simulink model "CrCtl_ShOff"  (R2016b)
settings: configuration reference "CodeGenConfigSet" (kept outside this file)
values from neighbouring files (symbols this model uses):
  CrCtl_aAccShOff_C = Calibration.Parameter    [init_CrCtl_ShOff.m]
  CrCtl_aDeclShOff_C = Calibration.Parameter    [init_CrCtl_ShOff.m]
  CrCtl_facDvtRelShOff_C = Calibration.Parameter    [init_CrCtl_ShOff.m]
  CrCtl_GearMin_C = Calibration.Parameter    [init_CrCtl_ShOff.m]
  CrCtl_nMaxShOff_C = Calibration.Parameter    [init_CrCtl_ShOff.m]
  CrCtl_nMinShOff_C = Calibration.Parameter    [init_CrCtl_ShOff.m]
  CRCTL_PAUSEENABLE_SY = uint8(0)    [init_CrCtl_ShOff.m]
  CrCtl_rTraV2NDvtAbsShOff_C = Calibration.Parameter    [init_CrCtl_ShOff.m]
  CrCtl_rTraV2NDvtShOff_C = Calibration.Parameter    [init_CrCtl_ShOff.m]
  CrCtl_rTraV2NSuspSync_C = Calibration.Parameter    [init_CrCtl_ShOff.m]
  CrCtl_stShOffCut_C = Calibration.Parameter    [init_CrCtl_ShOff.m]
  CrCtl_stShOffIrvrs_C = Calibration.Parameter    [init_CrCtl_ShOff.m]
  CrCtl_stShOffRvrs_C = Calibration.Parameter    [init_CrCtl_ShOff.m]
  CrCtl_stShOffRvrsDelVel_C = Calibration.Parameter    [init_CrCtl_ShOff.m]
  CrCtl_stShOffSlpCnstRmp_C = Calibration.Parameter    [init_CrCtl_ShOff.m]
  CrCtl_stShOffTimeCnstRmp_C = Calibration.Parameter    [init_CrCtl_ShOff.m]
  CrCtl_swtSuspEna_C = Calibration.Parameter    [init_CrCtl_ShOff.m]
  CrCtl_tiAccShOff_C = Calibration.Parameter    [init_CrCtl_ShOff.m]
  CrCtl_tiDeclShOff_C = Calibration.Parameter    [init_CrCtl_ShOff.m]
  CrCtl_tiDvtShOff_C = Calibration.Parameter    [init_CrCtl_ShOff.m]
  CrCtl_tiOverrideShOff_C = Calibration.Parameter    [init_CrCtl_ShOff.m]
  CrCtl_tiSuspClthPresMax_C = Calibration.Parameter    [init_CrCtl_ShOff.m]
  CrCtl_tiSuspMax_C = Calibration.Parameter    [init_CrCtl_ShOff.m]
  CrCtl_tiSuspSync_C = Calibration.Parameter    [init_CrCtl_ShOff.m]
  CrCtl_trqSpdGovInc_C = Calibration.Parameter    [init_CrCtl_ShOff.m]
  CrCtl_trqSpdGovMax_C = Calibration.Parameter    [init_CrCtl_ShOff.m]
  CrCtl_trqSpdGovRed_C = Calibration.Parameter    [init_CrCtl_ShOff.m]
  CrCtl_vDvtNegShOff_C = Calibration.Parameter    [init_CrCtl_ShOff.m]
  CrCtl_vDvtPosShOff_C = Calibration.Parameter    [init_CrCtl_ShOff.m]
  CrCtl_vDvtShOff_C = Calibration.Parameter    [init_CrCtl_ShOff.m]
  CrCtl_vMaxShOff_C = Calibration.Parameter    [init_CrCtl_ShOff.m]
  CrCtl_vMinShOff_C = Calibration.Parameter    [init_CrCtl_ShOff.m]
  TRQ_ENGINTV_SY = uint8(1)    [init_CrCtl_ShOff.m]
  VEL_ZERO = fi(0,VehSpeed_km_h)    [init_CrCtl_ShOff.m]
undefined symbols (not defined in the file or in its folder): CrCtl_ShOff_DT, CrCtl_stLck_conv, CrCtl_stOpFunc_conv, CrCtl_stShOff_conv, CrCtl_stSub_conv, CrCUI_BttnState_conv, CruiseCtl_State_conv, EngState_conv, Switch_conv
libraries: simulink x80, CXLib x24
(part 1 of 2)
settings Model: Creator=guanxiaoxing  LastModifiedBy=guanxiaoxing
settings ConfigSetRef: SourceLocation=Base Workspace

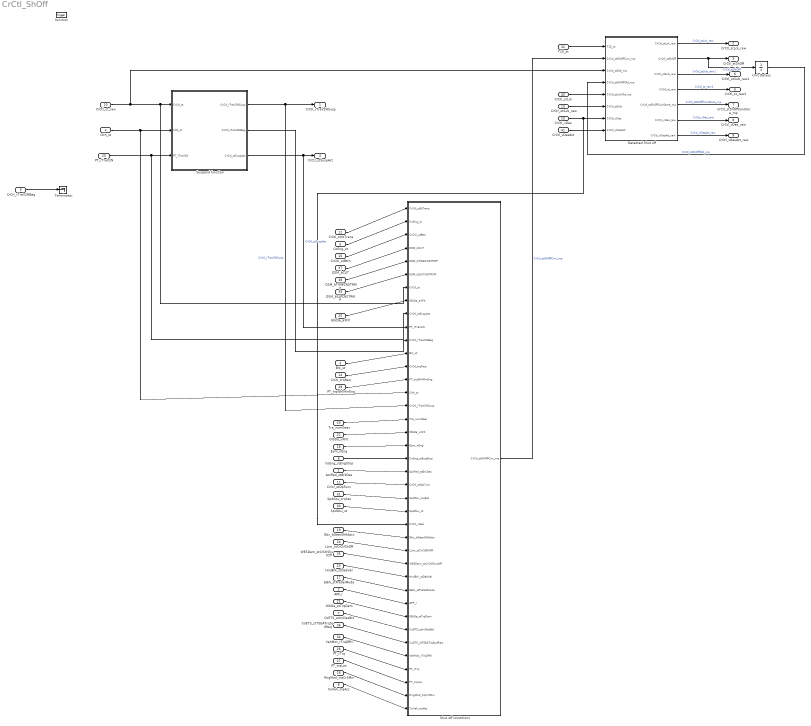
== system CrCtl_ShOff ==
  AccPed_stBrkDes : Inport  Description=Application parameter for engine brake request  OutMin=0  OutMax=255  OutDataTypeStr=State_uint8
  APP_r : Inport  Tag=%  Description=Acceleration pedal sensor 1 value after fault handling  Port=2  OutMin=0  OutMax=100  OutDataTypeStr=Accpedal_rate
  Brk_st : Inport  Description=Brake switch state  Port=3  OutMin=0  OutMax=255  OutDataTypeStr=State_uint8
  Clth_st : Inport  Description=Clutch information  Port=4  OutMin=0  OutMax=255  OutDataTypeStr=State_uint8
  CoEng_st : Inport  Description=Engine coordinator state  Port=5  OutDataTypeStr=Enum: EngState_conv
  CoEng_stEngStop : Inport  Description=Bit coded output message from engine stop function for low idle, egine shut off and crank control  Port=6  OutMin=0  OutMax=255  OutDataTypeStr=State_uint8
  CoETS_stInrDesBrk : Inport  Description=Negative torque status for inner torque  Port=7  OutMin=0  OutMax=4294967295  OutDataTypeStr=State_uint32
  CoVeh_trqAcs : Inport  Tag=Nm  Description=message for torque demand of accessories  Port=8  OutMin=-3276.8  OutMax=3276.7  OutDataTypeStr=Trq_Nm
  CrCtl_rTraV2NBeg : Inport  Tag=km/h/rpm  Description=V/N ratio at activation of cruise control  Port=9  OutMin=-0.32768  OutMax=0.32767  OutDataTypeStr=Tra_V2N_km_h_rpm
  CrCtl_st_raw : Inport  Description=Application parameter for Cruise Control state  Port=10  OutDataTypeStr=Enum: CruiseCtl_State_conv
  CrCtl_stOpFunc : Inport  Description=state of cruise control operation functionality  Port=11  OutDataTypeStr=Enum: CrCtl_stOpFunc_conv
  CrCtl_stStTrans : Inport  Description=|  Port=12  OutDataTypeStr=Enum: CrCUI_BttnState_conv
      | State transition demand to the state machine of
      | cruise control
  CrCtl_stSub_raw : Inport  Description=Cruise control sub mode  Port=13  OutDataTypeStr=Enum: CrCtl_stSub_conv
  CrCtl_trqReq : Inport  Tag=Nm  Description=Cruise control torque request  Port=14  OutMin=-3000  OutMax=3000  OutDataTypeStr=Trq_Nm
  CrCtl_vDes : Inport  Tag=km/h  Description=Cruise Control desired set point speed  Port=15  OutMin=0  OutMax=250  OutDataTypeStr=VehSpeed_km_h
  CrCUI_stBttn : Inport  Description=Application parameter for status button information  Port=16  OutDataTypeStr=Enum: CrCUI_BttnState_conv
  EBrk_stPreSelMode : Inport  Description=Status of Engine Brake Pre-Selection modes  Port=17  OutDataTypeStr=Enum: EBrk_stPreSelMode_conv
  Epm_nEng : Inport  Tag=rpm  Description=Engine speed  Port=18  OutMin=0  OutMax=6000  OutDataTypeStr=EngSpeed_rpm
  Gbx_bGearShftActv : Inport  Description=Status gear shift active  Port=19  OutMin=0  OutMax=1  OutDataTypeStr=boolean
  GlbDa_aXFlt : Inport  Tag=m/s^2  Description=Vehicle longitudinal acceleration filtered  Port=20  OutMin=-32  OutMax=32  OutDataTypeStr=Acc_m_s2
  GlbDa_stTrqDem : Inport  Description=Contains highest prior function with torque demand  Port=21  OutMin=0  OutMax=4294967295  OutDataTypeStr=State_uint32
  GlbDa_vXFlt : Inport  Tag=km/h  Description=Vehicle velocity filtered  Port=22  OutMin=0  OutMax=250  OutDataTypeStr=VehSpeed_km_h
  HndBrk_stDebVal : Inport  Description=Debounced value of Hand Brake switch  Port=23  OutMin=0  OutMax=255  OutDataTypeStr=State_uint8
  LLim_stCrCtlShOff : Inport  Description=shutoff request for cruise control  Port=24  OutMin=0  OutMax=1  OutDataTypeStr=boolean
  PT_rTraV2N : Inport  Tag=km/h/rpm  Description=Quotient of velocity and engine speed  Port=25  OutMin=-0.32768  OutMax=0.32767  OutDataTypeStr=Tra_V2N_km_h_rpm
  PT_rTrq : Inport  Description=Powertrain torque ratio  Port=26  OutMin=-100  OutMax=100  OutDataTypeStr=TransRatio
  PT_trqLos : Inport  Tag=Nm  Description=Parameter for loss torque of the drive train  Port=27  OutMin=-3000  OutMax=3000  OutDataTypeStr=Trq_Nm
  PT_trqWhlMinEng : Inport  Tag=Nm  Description=Minimum wheel torque from the engine  Port=28  OutMin=-3000  OutMax=3000  OutDataTypeStr=Trq_Nm
  RngMod_trqCrSMin : Inport  Tag=Nm  Description=Minimal crankshaft torque  Port=29  OutMin=-3276.8  OutMax=3276.7  OutDataTypeStr=Trq_Nm
  SpdGov_st : Inport  Description=Status speed control SpdGov  Port=30  OutMin=0  OutMax=65535  OutDataTypeStr=State_uint16
  SpdGov_trqSet : Inport  Tag=Nm  Description=Set point torque of the SpdGov on the fuel path  Port=31  OutMin=-3000  OutMax=3000  OutDataTypeStr=Trq_Nm
  T15_st : Inport  Description=Terminal 15 status after denouncing  Port=32  OutDataTypeStr=Enum: Switch_conv
  Tra_numGear : Inport  Description=Current gear information  Port=33  OutMin=-128  OutMax=127  OutDataTypeStr=Tra_num
  VehMot_rTrqDfftl : Inport  Description=Torque ratio of differential  Port=34  OutMin=-300  OutMax=300  OutDataTypeStr=TransRatio
  WESDem_stCrCtlShutOff : Inport  Description=Shut off of the cruise control  Port=35  OutMin=0  OutMax=1  OutDataTypeStr=boolean
  CoETS_stTSEATrqSpdReq : Inport  Description=Status of information about torque and speed intervention  Port=36  OutMin=0  OutMax=65535  OutDataTypeStr=State_uint16
  DSM_bCUT : Inport  Description=status of Fid_CUT  Port=37  OutMin=0  OutMax=1  OutDataTypeStr=boolean
  DSM_bTIMECNSTRMP : Inport  Description=status of Fid_TIMECNSTRMP  Port=38  OutMin=0  OutMax=1  OutDataTypeStr=boolean
  DSM_bSLPCNSTRMP : Inport  Description=status of Fid_SLPCNSTRMP  Port=39  OutMin=0  OutMax=1  OutDataTypeStr=boolean
  CrCtl_stLck : Inport  Description=Cruise Control lock Status  Port=40  OutDataTypeStr=Enum: CrCtl_stLck_conv
  CrCtl_vDesAct : Inport  Tag=km/h  Description=Target speed for cruise control  Port=41  OutMin=0  OutMax=250  OutDataTypeStr=VehSpeed_km_h
  function : TriggerPort  TriggerType=function-call  VariantControl=Variant
  Detected Shut off : Subsystem
  Shut off conditions : Subsystem
  Suspend function : Subsystem
  Terminator : Terminator
  Unit Delay1 : UnitDelay  InitialCondition=CrCtl_stShOff_conv.CRCTL_NOSHOFFCONACTV  SampleTime=-1
  CrCtl_rTraV2NSusp : Outport  Tag=km/h/rpm  Description=V/N ratio for the pressed clutch during active Suspend mode  OutMin=-0.32768  OutMax=0.32767  OutDataTypeStr=Tra_V2N_km_h_rpm
  CrCtl_stLck_raw : Outport  Description=Cruise Control lock Status  Port=2  OutDataTypeStr=Enum: CrCtl_stLck_conv
  CrCtl_stShOff : Outport  Description=cruise control shut-off requirement  Port=3  OutDataTypeStr=Enum: CrCtl_stShOff_conv
  CrCtl_stSuspAct : Outport  Description=Cruise Control suspend mode active Status  Port=4  OutMin=0  OutMax=1  OutDataTypeStr=boolean
  CrCtl_st_raw1 : Outport  Description=Application parameter for Cruise Control state  Port=5  OutDataTypeStr=Enum: CruiseCtl_State_conv
  CrCtl_stSub_raw1 : Outport  Description=Cruise control sub mode  Port=6  OutDataTypeStr=Enum: CrCtl_stSub_conv
  CrCtl_stShOffConStore_mp : Outport  Description=Status of Shutoff condition  Port=7  OutMin=0  OutMax=4294967295  OutDataTypeStr=State_uint32
  CrCtl_vDes_raw : Outport  Tag=km/h  Description=Cruise Control desired set point speed  Port=8  OutMin=0  OutMax=250  OutDataTypeStr=VehSpeed_km_h
  CrCtl_vDesAct_raw : Outport  Tag=km/h  Description=Target speed for cruise control  Port=9  OutMin=0  OutMax=250  OutDataTypeStr=VehSpeed_km_h
  wires:
  Suspend function/1(CrCtl_rTraV2NSusp) -> CrCtl_rTraV2NSusp/1, Shut off conditions/16(CrCtl_rTraV2NSusp)  "CrCtl_rTraV2NSusp"
  Detected Shut off/1(CrCtl_stLck_raw) -> CrCtl_stLck_raw/1  "CrCtl_stLck_raw"
  Detected Shut off/2(CrCtl_stShOff) -> Unit Delay1/1, CrCtl_stShOff/1  "CrCtl_stShOff"
  Suspend function/3(CrCtl_stSuspAct) -> CrCtl_stSuspAct/1, Shut off conditions/9(CrCtl_stSuspAct)  "CrCtl_stSuspAct"
  T15_st/1 -> Detected Shut off/1(T15_st)
  CrCtl_st_raw/1 -> Shut off conditions/7(CrCtl_st), Suspend function/1(CrCtl_st), Detected Shut off/3(CrCtl_stOld_mp)
  Shut off conditions/1(CrCtl_stShOffCon_mp) -> Detected Shut off/2(CrCtl_stShOffCon_mp)  "CrCtl_stShOffCon_mp"
  Unit Delay1/1 -> Detected Shut off/4(CrCtl_stShOffOld_mp)  "CrCtl_stShOffOld_mp"
  CrCtl_stStTrans/1 -> Shut off conditions/1(CrCtl_stStTrans)
  CoEng_st/1 -> Shut off conditions/2(CoEng_st)
  CrCUI_stBttn/1 -> Shut off conditions/3(CrCUI_stBttn)
  GlbDa_aXFlt/1 -> Shut off conditions/8(GlbDa_aXFlt)
  PT_rTraV2N/1 -> Suspend function/3(PT_rTraV2N), Shut off conditions/10(PT_rTraV2N)
  Suspend function/2(CrCtl_rTraV2NBeg) -> Shut off conditions/11(CrCtl_rTraV2NBeg)
  Brk_st/1 -> Shut off conditions/12(Brk_st)
  CrCtl_trqReq/1 -> Shut off conditions/13(CrCtl_trqReq)
  PT_trqWhlMinEng/1 -> Shut off conditions/14(PT_trqWhlMinEng)
  Clth_st/1 -> Shut off conditions/15(Clth_st), Suspend function/2(Clth_st)
  Tra_numGear/1 -> Shut off conditions/17(Tra_numGear)
  GlbDa_vXFlt/1 -> Shut off conditions/18(GlbDa_vXFlt)
  Epm_nEng/1 -> Shut off conditions/19(Epm_nEng)
  CoEng_stEngStop/1 -> Shut off conditions/20(CoEng_stEngStop)
  AccPed_stBrkDes/1 -> Shut off conditions/21(AccPed_stBrkDes)
  CrCtl_stOpFunc/1 -> Shut off conditions/22(CrCtl_stOpFunc)
  SpdGov_trqSet/1 -> Shut off conditions/23(SpdGov_trqSet)
  SpdGov_st/1 -> Shut off conditions/24(SpdGov_st)
  CrCtl_vDes/1 -> Shut off conditions/25(CrCtl_vDes), Detected Shut off/7(CrCtl_vDes)
  Gbx_bGearShftActv/1 -> Shut off conditions/26(Gbx_bGearShftActv)
  LLim_stCrCtlShOff/1 -> Shut off conditions/27(LLim_stCrCtlShOff)
  WESDem_stCrCtlShutOff/1 -> Shut off conditions/28(WESDem_stCrCtlShutOff)
  HndBrk_stDebVal/1 -> Shut off conditions/29(HndBrk_stDebVal)
  CoETS_stTSEATrqSpdReq/1 -> Shut off conditions/34(CoETS_stTSEATrqSpdReq)
  EBrk_stPreSelMode/1 -> Shut off conditions/30(EBrk_stPreSelMode)
  APP_r/1 -> Shut off conditions/31(APP_r)
  PT_rTrq/1 -> Shut off conditions/36(PT_rTrq)
  PT_trqLos/1 -> Shut off conditions/37(PT_trqLos)
  RngMod_trqCrSMin/1 -> Shut off conditions/38(RngMod_trqCrSMin)
  CoVeh_trqAcs/1 -> Shut off conditions/39(CoVeh_trqAcs)
  VehMot_rTrqDfftl/1 -> Shut off conditions/35(VehMot_rTrqDfftl)
  CoETS_stInrDesBrk/1 -> Shut off conditions/33(CoETS_stInrDesBrk)
  GlbDa_stTrqDem/1 -> Shut off conditions/32(GlbDa_stTrqDem)
  DSM_bCUT/1 -> Shut off conditions/4(DSM_bCUT)
  DSM_bTIMECNSTRMP/1 -> Shut off conditions/5(DSM_bTIMECNSTRMP)
  DSM_bSLPCNSTRMP/1 -> Shut off conditions/6(DSM_bSLPCNSTRMP)
  CrCtl_stSub_raw/1 -> Detected Shut off/6(CrCtl_stSub)
  Detected Shut off/5(CrCtl_stShOffConStore_mp) -> CrCtl_stShOffConStore_mp/1  "CrCtl_stShOffConStore_mp"
  CrCtl_rTraV2NBeg/1 -> Terminator/1
  CrCtl_stLck/1 -> Detected Shut off/5(CrCtl_stLckOld_mp)
  Detected Shut off/6(CrCtl_vDes_raw) -> CrCtl_vDes_raw/1  "CrCtl_vDes_raw"
  Detected Shut off/7(CrCtl_vDesAct_raw) -> CrCtl_vDesAct_raw/1  "CrCtl_vDesAct_raw"
  CrCtl_vDesAct/1 -> Detected Shut off/8(CrCtl_vDesAct)
  Detected Shut off/3(CrCtl_stSub_raw) -> CrCtl_stSub_raw1/1  "CrCtl_stSub_raw1"
  Detected Shut off/4(CrCtl_st_raw) -> CrCtl_st_raw1/1  "CrCtl_st_raw1"

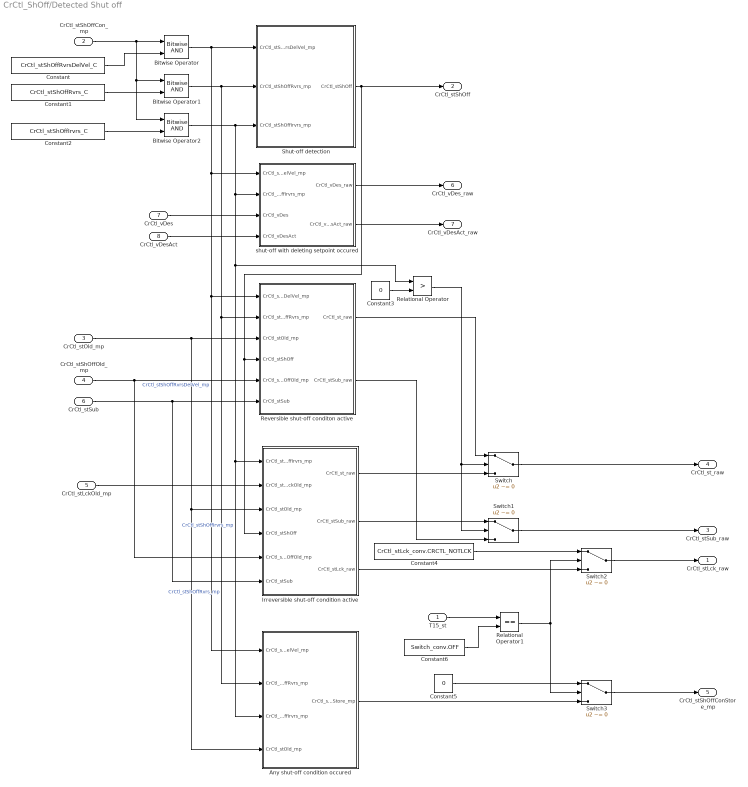
== system CrCtl_ShOff/Detected Shut off ==
  T15_st : Inport
  CrCtl_stShOffCon_mp : Inport  Port=2
  CrCtl_stOld_mp : Inport  Port=3
  CrCtl_stShOffOld_mp : Inport  Port=4
  CrCtl_stLckOld_mp : Inport  Port=5
  CrCtl_stSub : Inport  Port=6
  CrCtl_vDes : Inport  Port=7
  CrCtl_vDesAct : Inport  Port=8
  Any shut-off condition occured : Subsystem
  Bitwise Operator : simulink/Logic and Bit Operations/Bitwise Operator  logicop=AND  UseBitMask=off  NumInputPorts=2  BitMask=bin2dec('11011001')  BitMaskRealWorld=Stored Integer
  Bitwise Operator1 : simulink/Logic and Bit Operations/Bitwise Operator  logicop=AND  UseBitMask=off  NumInputPorts=2  BitMask=bin2dec('11011001')  BitMaskRealWorld=Stored Integer
  Bitwise Operator2 : simulink/Logic and Bit Operations/Bitwise Operator  logicop=AND  UseBitMask=off  NumInputPorts=2  BitMask=bin2dec('11011001')  BitMaskRealWorld=Stored Integer
  Constant : Constant  Value=CrCtl_stShOffRvrsDelVel_C
  Constant1 : Constant  Value=CrCtl_stShOffRvrs_C
  Constant2 : Constant  Value=CrCtl_stShOffIrvrs_C
  Constant3 : Constant  Value=0
  Constant4 : Constant  Value=CrCtl_stLck_conv.CRCTL_NOTLCK
  Constant5 : Constant  Value=0  OutDataTypeStr=uint16
  Constant6 : Constant  Value=Switch_conv.OFF
  Irreversible shut-off condition active : Subsystem
  Relational Operator : RelationalOperator  Operator=>  OutDataTypeStr=boolean  RndMeth=Simplest
  Relational Operator1 : RelationalOperator  Operator===  OutDataTypeStr=boolean  RndMeth=Simplest
  Reversible shut-off conditon active : Subsystem
  Shut-off detection : Subsystem
  Switch{,1..3} (4 alike) : Switch  Criteria=u2 ~= 0
  shut-off with deleting setpoint occured : Subsystem
  CrCtl_stLck_raw : Outport
  CrCtl_stShOff : Outport  Port=2
  CrCtl_stSub_raw : Outport  Port=3
  CrCtl_st_raw : Outport  Port=4
  CrCtl_stShOffConStore_mp : Outport  Port=5
  CrCtl_vDes_raw : Outport  Port=6
  CrCtl_vDesAct_raw : Outport  Port=7
  wires:
  CrCtl_stShOffCon_mp/1 -> Bitwise Operator2/1, Bitwise Operator1/1, Bitwise Operator/1
  Constant/1 -> Bitwise Operator/2
  Constant1/1 -> Bitwise Operator1/2
  Constant2/1 -> Bitwise Operator2/2
  Bitwise Operator/1 -> Shut-off detection/1(CrCtl_stShOffRvrsDelVel_mp), Any shut-off condition occured/1(CrCtl_stShOffRvrsDelVel_mp), Reversible shut-off conditon active/1(CrCtl_stShOffRvrsDelVel_mp), shut-off with deleting setpoint occured/1(CrCtl_stShOffRvrsDelVel_mp)  "CrCtl_stShOffRvrsDelVel_mp"
  Bitwise Operator1/1 -> Any shut-off condition occured/2(CrCtl_stShOffRvrs_mp), Reversible shut-off conditon active/2(CrCtl_stShOffRvrs_mp), Shut-off detection/2(CrCtl_stShOffRvrs_mp)  "CrCtl_stShOffRvrs_mp"
  Bitwise Operator2/1 -> Relational Operator/1, Irreversible shut-off condition active/1(CrCtl_stShOffIrvrs_mp), Any shut-off condition occured/3(CrCtl_stShOffIrvrs_mp), shut-off with deleting setpoint occured/2(CrCtl_stShOffIrvrs_mp), Shut-off detection/3(CrCtl_stShOffIrvrs_mp)  "CrCtl_stShOffIrvrs_mp"
  Constant3/1 -> Relational Operator/2
  CrCtl_stOld_mp/1 -> Any shut-off condition occured/4(CrCtl_stOld_mp), Irreversible shut-off condition active/3(CrCtl_stOld_mp), Reversible shut-off conditon active/3(CrCtl_stOld_mp)
  CrCtl_stShOffOld_mp/1 -> Irreversible shut-off condition active/5(CrCtl_stShOffOld_mp), Reversible shut-off conditon active/5(CrCtl_stShOffOld_mp)
  Reversible shut-off conditon active/1(CrCtl_st_raw) -> Switch/1
  Relational Operator/1 -> Switch/2, Switch1/2
  Irreversible shut-off condition active/1(CrCtl_st_raw) -> Switch/3
  Reversible shut-off conditon active/2(CrCtl_stSub_raw) -> Switch1/3
  Irreversible shut-off condition active/3(CrCtl_stLck_raw) -> Switch2/3
  Irreversible shut-off condition active/2(CrCtl_stSub_raw) -> Switch1/1
  Relational Operator1/1 -> Switch3/2, Switch2/2
  Constant4/1 -> Switch2/1
  Any shut-off condition occured/1(CrCtl_stShOffConStore_mp) -> Switch3/3
  Constant5/1 -> Switch3/1
  Switch1/1 -> CrCtl_stSub_raw/1
  Switch/1 -> CrCtl_st_raw/1
  Switch3/1 -> CrCtl_stShOffConStore_mp/1
  shut-off with deleting setpoint occured/1(CrCtl_vDes_raw) -> CrCtl_vDes_raw/1
  Switch2/1 -> CrCtl_stLck_raw/1
  Shut-off detection/1(CrCtl_stShOff) -> CrCtl_stShOff/1, Irreversible shut-off condition active/4(CrCtl_stShOff), Reversible shut-off conditon active/4(CrCtl_stShOff)
  CrCtl_stSub/1 -> Irreversible shut-off condition active/6(CrCtl_stSub), Reversible shut-off conditon active/6(CrCtl_stSub)
  CrCtl_stLckOld_mp/1 -> Irreversible shut-off condition active/2(CrCtl_stLckOld_mp)
  CrCtl_vDes/1 -> shut-off with deleting setpoint occured/3(CrCtl_vDes)
  shut-off with deleting setpoint occured/2(CrCtl_vDesAct_raw) -> CrCtl_vDesAct_raw/1
  CrCtl_vDesAct/1 -> shut-off with deleting setpoint occured/4(CrCtl_vDesAct)
  T15_st/1 -> Relational Operator1/1
  Constant6/1 -> Relational Operator1/2

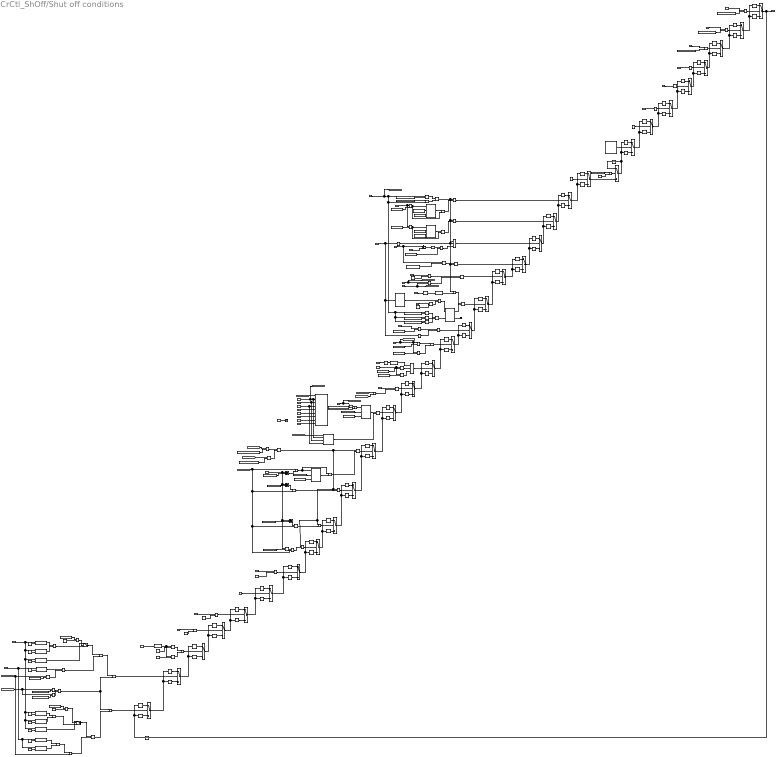
== system CrCtl_ShOff/Shut off conditions ==
  CrCtl_stStTrans : Inport
  CoEng_st : Inport  Port=2
  CrCUI_stBttn : Inport  Port=3
  DSM_bCUT : Inport  Port=4
  DSM_bTIMECNSTRMP : Inport  Port=5
  DSM_bSLPCNSTRMP : Inport  Port=6
  CrCtl_st : Inport  Port=7
  GlbDa_aXFlt : Inport  Port=8
  CrCtl_stSuspAct : Inport  Port=9
  PT_rTraV2N : Inport  Port=10
  CrCtl_rTraV2NBeg : Inport  Port=11
  Brk_st : Inport  Port=12
  CrCtl_trqReq : Inport  Port=13
  PT_trqWhlMinEng : Inport  Port=14
  Clth_st : Inport  Port=15
  CrCtl_rTraV2NSusp : Inport  Port=16
  Tra_numGear : Inport  Port=17
  GlbDa_vXFlt : Inport  Port=18
  Epm_nEng : Inport  Port=19
  CoEng_stEngStop : Inport  Port=20
  AccPed_stBrkDes : Inport  Port=21
  CrCtl_stOpFunc : Inport  Port=22
  SpdGov_trqSet : Inport  Port=23
  SpdGov_st : Inport  Port=24
  CrCtl_vDes : Inport  Port=25
  Gbx_bGearShftActv : Inport  Port=26
  LLim_stCrCtlShOff : Inport  Port=27
  WESDem_stCrCtlShutOff : Inport  Port=28
  HndBrk_stDebVal : Inport  Port=29
  EBrk_stPreSelMode : Inport  Port=30
  APP_r : Inport  Port=31
  GlbDa_stTrqDem : Inport  Port=32
  CoETS_stInrDesBrk : Inport  Port=33
  CoETS_stTSEATrqSpdReq : Inport  Port=34
  VehMot_rTrqDfftl : Inport  Port=35
  PT_rTrq : Inport  Port=36
  PT_trqLos : Inport  Port=37
  RngMod_trqCrSMin : Inport  Port=38
  CoVeh_trqAcs : Inport  Port=39
  Abs : Abs
  Add : Sum  Inputs=+-
  Add1 : Sum
  Add2 : Sum
  Add3 : Sum  Inputs=+-
  Bit Clear : simulink/Logic and Bit Operations/Bit Clear  iBit=0
  Bit Clear1 : simulink/Logic and Bit Operations/Bit Clear  iBit=1
  Bit Clear10 : simulink/Logic and Bit Operations/Bit Clear  iBit=11
  Bit Clear11 : simulink/Logic and Bit Operations/Bit Clear  iBit=12
  Bit Clear12 : simulink/Logic and Bit Operations/Bit Clear  iBit=13
  Bit Clear13 : simulink/Logic and Bit Operations/Bit Clear  iBit=14
  Bit Clear14 : simulink/Logic and Bit Operations/Bit Clear  iBit=15
  Bit Clear15 : simulink/Logic and Bit Operations/Bit Clear  iBit=16
  Bit Clear16 : simulink/Logic and Bit Operations/Bit Clear  iBit=17
  Bit Clear17 : simulink/Logic and Bit Operations/Bit Clear  iBit=18
  Bit Clear18 : simulink/Logic and Bit Operations/Bit Clear  iBit=19
  Bit Clear19 : simulink/Logic and Bit Operations/Bit Clear  iBit=20
  Bit Clear2 : simulink/Logic and Bit Operations/Bit Clear  iBit=2
  Bit Clear20 : simulink/Logic and Bit Operations/Bit Clear  iBit=21
  Bit Clear21 : simulink/Logic and Bit Operations/Bit Clear  iBit=22
  Bit Clear22 : simulink/Logic and Bit Operations/Bit Clear  iBit=23
  Bit Clear23 : simulink/Logic and Bit Operations/Bit Clear  iBit=24
  Bit Clear24 : simulink/Logic and Bit Operations/Bit Clear  iBit=25
  Bit Clear25 : simulink/Logic and Bit Operations/Bit Clear  iBit=26
  Bit Clear26 : simulink/Logic and Bit Operations/Bit Clear  iBit=27
  Bit Clear27 : simulink/Logic and Bit Operations/Bit Clear  iBit=28
  Bit Clear28 : simulink/Logic and Bit Operations/Bit Clear  iBit=29
  Bit Clear29 : simulink/Logic and Bit Operations/Bit Clear  iBit=30
  Bit Clear3 : simulink/Logic and Bit Operations/Bit Clear  iBit=3
  Bit Clear30 : simulink/Logic and Bit Operations/Bit Clear  iBit=31
  Bit Clear4 : simulink/Logic and Bit Operations/Bit Clear  iBit=4
  Bit Clear5 : simulink/Logic and Bit Operations/Bit Clear  iBit=5
  Bit Clear6 : simulink/Logic and Bit Operations/Bit Clear  iBit=6
  Bit Clear7 : simulink/Logic and Bit Operations/Bit Clear  iBit=7
  Bit Clear8 : simulink/Logic and Bit Operations/Bit Clear  iBit=8
  Bit Clear9 : simulink/Logic and Bit Operations/Bit Clear  iBit=10
  Bit Set : simulink/Logic and Bit Operations/Bit Set  iBit=0
  Bit Set1 : simulink/Logic and Bit Operations/Bit Set  iBit=1
  Bit Set10 : simulink/Logic and Bit Operations/Bit Set  iBit=11
  Bit Set11 : simulink/Logic and Bit Operations/Bit Set  iBit=12
  Bit Set12 : simulink/Logic and Bit Operations/Bit Set  iBit=13
  Bit Set13 : simulink/Logic and Bit Operations/Bit Set  iBit=14
  Bit Set14 : simulink/Logic and Bit Operations/Bit Set  iBit=15
  Bit Set15 : simulink/Logic and Bit Operations/Bit Set  iBit=16
  Bit Set16 : simulink/Logic and Bit Operations/Bit Set  iBit=17
  Bit Set17 : simulink/Logic and Bit Operations/Bit Set  iBit=18
  Bit Set18 : simulink/Logic and Bit Operations/Bit Set  iBit=19
  Bit Set19 : simulink/Logic and Bit Operations/Bit Set  iBit=20
  Bit Set2 : simulink/Logic and Bit Operations/Bit Set  iBit=2
  Bit Set20 : simulink/Logic and Bit Operations/Bit Set  iBit=21
  Bit Set21 : simulink/Logic and Bit Operations/Bit Set  iBit=22
  Bit Set22 : simulink/Logic and Bit Operations/Bit Set  iBit=23
  Bit Set23 : simulink/Logic and Bit Operations/Bit Set  iBit=24
  Bit Set24 : simulink/Logic and Bit Operations/Bit Set  iBit=25
  Bit Set25 : simulink/Logic and Bit Operations/Bit Set  iBit=26
  Bit Set26 : simulink/Logic and Bit Operations/Bit Set  iBit=27
  Bit Set27 : simulink/Logic and Bit Operations/Bit Set  iBit=28
  Bit Set28 : simulink/Logic and Bit Operations/Bit Set  iBit=29
  Bit Set29 : simulink/Logic and Bit Operations/Bit Set  iBit=30
  Bit Set3 : simulink/Logic and Bit Operations/Bit Set  iBit=3
  Bit Set30 : simulink/Logic and Bit Operations/Bit Set  iBit=31
  Bit Set4 : simulink/Logic and Bit Operations/Bit Set  iBit=4
  Bit Set5 : simulink/Logic and Bit Operations/Bit Set  iBit=5
  Bit Set6 : simulink/Logic and Bit Operations/Bit Set  iBit=6
  Bit Set7 : simulink/Logic and Bit Operations/Bit Set  iBit=7
  Bit Set8 : simulink/Logic and Bit Operations/Bit Set  iBit=8
  Bit Set9 : simulink/Logic and Bit Operations/Bit Set  iBit=10
  Bitwise Operator1 : simulink/Logic and Bit Operations/Bitwise Operator  logicop=AND  UseBitMask=on  BitMask=bin2dec('00000001')  BitMaskRealWorld=Stored Integer
  Bitwise Operator2 : simulink/Logic and Bit Operations/Bitwise Operator  logicop=AND  UseBitMask=on  BitMask=bin2dec('00000010')  BitMaskRealWorld=Stored Integer
  Chk_DrvDemActv : Subsystem
  Chk_DrvDemActv_Hi : Subsystem
  Constant : Constant  Value=CrCUI_BttnState_conv.CRCUI_SWTOFF
  Constant1 : Constant  Value=EngState_conv.COENG_RUNNING
  Constant{10,12,28,32} (4 alike) : Constant  Value=CrCtl_ShOff_DT
  Constant11 : Constant  Value=CrCtl_aDeclShOff_C
  Constant13 : Constant  Value=CrCtl_tiAccShOff_C
  Constant14 : Constant  Value=CrCtl_aAccShOff_C
  Constant15 : Constant  Value=CrCtl_rTraV2NDvtShOff_C
  Constant16 : Constant  Value=CrCtl_rTraV2NDvtAbsShOff_C
  Constant17 : Constant  OutDataTypeStr=uint8
  Constant18 : Constant  Value=0.0  OutDataTypeStr=Tra_V2N_km_h_rpm
  Constant2 : Constant  Value=CrCUI_BttnState_conv.CRCUI_MODEERR
  Constant20 : Constant  Value=CruiseCtl_State_conv.CrCtl_ERROR
  Constant21 : Constant  Value=CrCtl_GearMin_C
  Constant22 : Constant  Value=CrCtl_vMaxShOff_C
  Constant23 : Constant  Value=CrCtl_vMinShOff_C
  Constant24 : Constant  Value=CrCtl_nMaxShOff_C
  Constant25 : Constant  Value=CrCtl_nMinShOff_C
  Constant26 : Constant  Value=CrCtl_stOpFunc_conv.CRCTL_OVERRIDE
  Constant27 : Constant  Value=CrCtl_tiOverrideShOff_C
  Constant29 : Constant  Value=CruiseCtl_State_conv.CrCtl_CRUISE
  Constant{3..4,38..39,49,55} (6 alike) : Constant  Value=0
  Constant30 : Constant  Value=CrCtl_stOpFunc_conv.CRCTL_ACTV
  Constant31 : Constant  Value=CrCtl_tiDvtShOff_C
  Constant33 : Constant  Value=CrCtl_vDvtShOff_C
  Constant34 : Constant  Value=CrCtl_vDvtPosShOff_C
  Constant35 : Constant  Value=CrCtl_vDvtNegShOff_C
  Constant36 : Constant  Value=CrCtl_facDvtRelShOff_C
  Constant37 : Constant  Value=true
  Constant40 : Constant  Value=3  OutDataTypeStr=uint8
  Constant41 : Constant  Value=5  OutDataTypeStr=uint8
  Constant42 : Constant  Value=5  OutDataTypeStr=uint8
  Constant43 : Constant  OutDataTypeStr=uint8
  Constant44 : Constant  Value=16  OutDataTypeStr=uint8
  Constant45 : Constant  Value=2  OutDataTypeStr=uint8
  Constant46 : Constant  Value=4  OutDataTypeStr=uint8
  Constant47 : Constant  Value=17  OutDataTypeStr=uint8
  Constant48 : Constant  Value=TRQ_ENGINTV_SY
  Constant5 : Constant  Value=CruiseCtl_State_conv.CrCtl_STAND_BY
  Constant50 : Constant  Value=11  OutDataTypeStr=uint8
  Constant51 : Constant  Value=CrCtl_trqSpdGovMax_C
  Constant52 : Constant  Value=CruiseCtl_State_conv.CrCtl_OFF
  Constant53 : Constant  Value=CruiseCtl_State_conv.CrCtl_STAND_BY
  Constant54 : Constant  Value=TRQ_ENGINTV_SY
  Constant56 : Constant  Value=10  OutDataTypeStr=uint8
  Constant57 : Constant  Value=11  OutDataTypeStr=uint8
  Constant58 : Constant  Value=CruiseCtl_State_conv.CrCtl_STAND_BY
  Constant59 : Constant  Value=CruiseCtl_State_conv.CrCtl_OFF
  Constant6 : Constant  Value=CRCTL_PAUSEENABLE_SY
  Constant7 : Constant
  Constant8 : Constant  Value=CruiseCtl_State_conv.CrCtl_OFF
  Constant9 : Constant  Value=CrCtl_tiDeclShOff_C
  Data Type Conversion : DataTypeConversion  OutDataTypeStr=boolean
  Data Type Conversion1 : DataTypeConversion  OutDataTypeStr=boolean
  Data Type Conversion2 : DataTypeConversion  OutDataTypeStr=uint8
  EBC1/VDC1 Shut off conditons : Subsystem
  EdgeFalling : CXLib/EdgeFalling
  GetBit{,1..5} (6 alike) : CXLib/GetBit  dataTypeString=uint32  dataLength=0
      settings: AttributesFormatString=Get bit from %<dataTypeString>
  GetBit6 : CXLib/GetBit  dataTypeString=uint16  dataLength=0
      settings: AttributesFormatString=Get bit from %<dataTypeString>
  GetBit7 : CXLib/GetBit  dataTypeString=uint16  dataLength=0
      settings: AttributesFormatString=Get bit from %<dataTypeString>
  GetBit8 : CXLib/GetBit  dataTypeString=uint16  dataLength=0
      settings: AttributesFormatString=Get bit from %<dataTypeString>
  Logical Operator{,1..2,8,17} (5 alike) : Logic  Operator=NOT  AllPortsSameDT=off  OutDataTypeStr=boolean
  Logical Operator{3..7,10..12,14,16,20,23..28,32..34,37..39} (23 alike) : Logic  AllPortsSameDT=off  OutDataTypeStr=boolean
  Logical Operator{13,18,21..22,29..31,35..36} (9 alike) : Logic  Operator=OR  AllPortsSameDT=off  OutDataTypeStr=boolean
  Logical Operator15 : Logic  Operator=OR  Inputs=3  AllPortsSameDT=off  OutDataTypeStr=boolean
  Logical Operator19 : Logic  Operator=OR  Inputs=3  AllPortsSameDT=off  OutDataTypeStr=boolean
  Logical Operator9 : Logic  Inputs=3  AllPortsSameDT=off  OutDataTypeStr=boolean
  Product : Product
  RSFlipFlop : CXLib/RSFlipFlop
  Relational Operator{,2,4,6..7,14,20,22,24,28..29,31..32,38} (14 alike) : RelationalOperator  Operator===  OutDataTypeStr=boolean  RndMeth=Simplest
  Relational Operator{1,3,5,12,33,35..37} (8 alike) : RelationalOperator  Operator=~=  OutDataTypeStr=boolean  RndMeth=Simplest
  Relational Operator{9..10,19,23,27,30,34} (7 alike) : RelationalOperator  Operator=>  OutDataTypeStr=boolean  RndMeth=Simplest
  Relational Operator{8,11,15,18} (4 alike) : RelationalOperator  Operator=<  OutDataTypeStr=boolean  RndMeth=Simplest
  Relational Operator{13,17,21,26} (4 alike) : RelationalOperator  OutDataTypeStr=boolean  RndMeth=Simplest
  Relational Operator16 : RelationalOperator  Operator=<=  OutDataTypeStr=boolean  RndMeth=Simplest
  Relational Operator25 : RelationalOperator  Operator=<=  OutDataTypeStr=boolean  RndMeth=Simplest
  Switch{,1..33} (34 alike) : Switch  Criteria=u2 ~= 0
  Terminator : Terminator
  Terminator1 : Terminator
  TurnOnDelay{,1..3} (4 alike) : CXLib/TurnOnDelay
  Unit Delay : UnitDelay  SampleTime=-1
  Unit Delay1 : UnitDelay  SampleTime=-1
  CrCtl_stShOffCon_mp : Outport
  wires:
  CrCtl_stStTrans/1 -> Relational Operator/1
  Constant/1 -> Relational Operator/2
  Bit Set/1 -> Switch/1
  Bit Clear/1 -> Switch/3
  Switch1/1 -> Bit Clear/1, Bit Set/1
  CoEng_st/1 -> Relational Operator1/1
  Constant1/1 -> Relational Operator1/2
  Bit Set1/1 -> Switch1/1
  Bit Clear1/1 -> Switch1/3
  Switch2/1 -> Bit Clear1/1, Bit Set1/1
  CrCUI_stBttn/1 -> Relational Operator2/1
  Constant2/1 -> Relational Operator2/2
  Bit Set2/1 -> Switch2/1
  Bit Clear2/1 -> Switch2/3
  Switch3/1 -> Bit Clear2/1, Bit Set2/1
  Bit Set3/1 -> Switch3/1
  Bit Clear3/1 -> Switch3/3
  Switch4/1 -> Bit Clear3/1, Bit Set3/1
  DSM_bCUT/1 -> Logical Operator/1
  Bit Clear4/1 -> Switch4/3
  Switch5/1 -> Bit Set4/1, Bit Clear4/1
  DSM_bTIMECNSTRMP/1 -> Logical Operator1/1
  Bit Set4/1 -> Switch4/1
  Bit Clear5/1 -> Switch5/3
  Switch6/1 -> Bit Set5/1, Bit Clear5/1
  DSM_bSLPCNSTRMP/1 -> Logical Operator2/1
  Bit Set5/1 -> Switch5/1
  Bit Clear6/1 -> Switch6/3
  Switch7/1 -> Bit Set6/1, Bit Clear6/1
  Bit Set6/1 -> Switch6/1
  Bit Clear7/1 -> Switch7/3
  Bit Set7/1 -> Switch7/1
  Switch9/1 -> Unit Delay1/1, Bit Clear7/1, Bit Set7/1
  Bit Clear8/1 -> Switch8/3
  Bit Set8/1 -> Switch8/1
  Switch10/1 -> Bit Clear8/1, Bit Set8/1
  Switch8/1 -> Switch9/3
  Constant6/1 -> Relational Operator4/1
  Constant7/1 -> Relational Operator4/2
  Relational Operator4/1 -> Switch9/2
  CrCtl_st/1 -> [CrCtl_st], Relational Operator3/1, Relational Operator5/2, Relational Operator38/1, Relational Operator6/1, Relational Operator7/1
  Constant5/1 -> Relational Operator3/2
  Constant8/1 -> Relational Operator5/1
  Relational Operator3/1 -> Logical Operator3/1
  Relational Operator5/1 -> Logical Operator3/2
  Constant9/1 -> TurnOnDelay/2
  Constant10/1 -> TurnOnDelay/3
  GlbDa_aXFlt/1 -> Relational Operator9/1, Relational Operator8/1
  Constant11/1 -> Relational Operator8/2
  Relational Operator8/1 -> Logical Operator4/2, TurnOnDelay/1
  TurnOnDelay/1 -> Logical Operator4/1
  Logical Operator3/1 -> Logical Operator9/1, Logical Operator7/1, Logical Operator5/1
  Logical Operator4/1 -> Logical Operator5/2
  Constant13/1 -> TurnOnDelay1/2
  Constant12/1 -> TurnOnDelay1/3
  Relational Operator9/1 -> TurnOnDelay1/1, Logical Operator6/2
  TurnOnDelay1/1 -> Logical Operator6/1
  Logical Operator6/1 -> Logical Operator7/2
  Constant14/1 -> Relational Operator9/2
  Bit Clear9/1 -> Switch10/3
  Bit Set9/1 -> Switch10/1
  Switch11/1 -> Bit Clear9/1, Bit Set9/1
  Bit Clear10/1 -> Switch11/3
  Bit Set10/1 -> Switch11/1
  Switch12/1 -> Bit Clear10/1, Bit Set10/1
  Logical Operator8/1 -> Logical Operator12/1, Logical Operator10/2, Logical Operator9/2
  PT_rTraV2N/1 -> Relational Operator11/1, Add/1
  CrCtl_rTraV2NBeg/1 -> Add/2
  Add/1 -> Abs/1
  Constant15/1 -> Relational Operator10/2
  Abs/1 -> Relational Operator10/1
  Relational Operator10/1 -> Logical Operator9/3
  Bit Clear11/1 -> Switch12/3
  Bit Set11/1 -> Switch12/1
  Switch13/1 -> Bit Clear11/1, Bit Set11/1
  Constant16/1 -> Relational Operator11/2
  Relational Operator11/1 -> Logical Operator10/1
  Bit Clear12/1 -> Switch13/3
  Bit Set12/1 -> Switch13/1
  Switch14/1 -> Bit Clear12/1, Bit Set12/1
  Brk_st/1 -> Relational Operator12/1
  Constant17/1 -> Relational Operator12/2
  Relational Operator12/1 -> Logical Operator11/1
  CrCtl_trqReq/1 -> [CrCtl_trqReq], Relational Operator13/1
  PT_trqWhlMinEng/1 -> Relational Operator13/2, [PT_trqWhlMinEng]
  Relational Operator13/1 -> Logical Operator11/2
  Bit Clear13/1 -> Switch14/3
  Bit Set13/1 -> Switch14/1
  Switch15/1 -> Bit Clear13/1, Bit Set13/1
  Clth_st/1 -> Bitwise Operator1/1
  Bitwise Operator1/1 -> Data Type Conversion/1
  Data Type Conversion/1 -> Logical Operator12/2
  Logical Operator12/1 -> Logical Operator13/1
  CrCtl_rTraV2NSusp/1 -> Relational Operator14/1
  Constant18/1 -> Relational Operator14/2
  Relational Operator14/1 -> Logical Operator14/2
  EdgeFalling/1 -> Logical Operator14/1
  Constant20/1 -> Relational Operator7/2
  Bit Clear14/1 -> Switch15/3
  Bit Set14/1 -> Switch15/1
  Switch16/1 -> Bit Clear14/1, Bit Set14/1
  RSFlipFlop/2 -> Terminator/1
  Relational Operator7/1 -> Logical Operator15/3
  Relational Operator38/1 -> Logical Operator15/1
  Logical Operator15/1 -> RSFlipFlop/2
  Logical Operator14/1 -> RSFlipFlop/1
  RSFlipFlop/1 -> Logical Operator13/2
  Tra_numGear/1 -> Relational Operator15/1
  Constant21/1 -> Relational Operator15/2
  Relational Operator15/1 -> Logical Operator16/1
  CrCtl_stSuspAct/1 -> Logical Operator17/1, EdgeFalling/1, Logical Operator8/1
  Logical Operator17/1 -> Logical Operator16/2
  Bit Clear15/1 -> Switch16/3
  Bit Set15/1 -> Switch16/1
  Switch17/1 -> Bit Clear15/1, Bit Set15/1
  Logical Operator16/1 -> Switch16/2
  GlbDa_vXFlt/1 -> [GlbDa_vXFlt], Relational Operator16/1, Relational Operator17/1
  Constant22/1 -> Relational Operator17/2
  Constant23/1 -> Relational Operator16/2
  Relational Operator17/1 -> Logical Operator18/1
  Relational Operator16/1 -> Logical Operator18/2
  Bit Clear16/1 -> Switch17/3
  Bit Set16/1 -> Switch17/1
  Switch18/1 -> Bit Clear16/1, Bit Set16/1
  Epm_nEng/1 -> Relational Operator18/1, Relational Operator19/1
  Constant24/1 -> Relational Operator19/2
  Constant25/1 -> Relational Operator18/2
  Relational Operator19/1 -> Logical Operator19/2
  Relational Operator18/1 -> Logical Operator19/3
  Bit Clear17/1 -> Switch18/3
  Bit Set17/1 -> Switch18/1
  Switch19/1 -> Bit Clear17/1, Bit Set17/1
  Bitwise Operator2/1 -> Data Type Conversion1/1
  Data Type Conversion1/1 -> Logical Operator19/1
  CoEng_stEngStop/1 -> Bitwise Operator2/1
  Bit Clear18/1 -> Switch19/3
  Bit Set18/1 -> Switch19/1
  Switch20/1 -> Bit Clear18/1, Bit Set18/1
  [PT_trqWhlMinEng] -> Relational Operator21/1
  AccPed_stBrkDes/1 -> Logical Operator20/1
  [CrCtl_trqReq] -> Relational Operator21/2
  Relational Operator21/1 -> Logical Operator20/2
  CrCtl_stOpFunc/1 -> [CrCtl_stOpFunc], Relational Operator20/1
  Constant26/1 -> Relational Operator20/2
  Relational Operator20/1 -> Logical Operator21/1
  Logical Operator21/1 -> TurnOnDelay2/1
  Constant27/1 -> TurnOnDelay2/2
  TurnOnDelay2/1 -> Logical Operator22/1
  Bit Clear19/1 -> Switch20/3
  Bit Set19/1 -> Switch20/1
  Switch21/1 -> Bit Clear19/1, Bit Set19/1
  SpdGov_st/1 -> Chk_DrvDemActv_Hi/3(SpdGov_st), Chk_DrvDemActv/3(SpdGov_st)
  SpdGov_trqSet/1 -> [SpdGov_trqSet], Chk_DrvDemActv_Hi/2(SpdGov_trqSet), Chk_DrvDemActv/2(SpdGov_trqSet)
  [CrCtl_trqReq] -> Chk_DrvDemActv/1(CrCtl_trqReq)
  Chk_DrvDemActv/1(Out1) -> Logical Operator21/2
  Constant28/1 -> TurnOnDelay2/3
  [CrCtl_st] -> Chk_DrvDemActv_Hi/1(CrCtl_st)
  Chk_DrvDemActv_Hi/1(Out1) -> Logical Operator22/2
  Bit Clear20/1 -> Switch21/3
  Bit Set20/1 -> Switch21/1
  Switch22/1 -> Bit Clear20/1, Bit Set20/1
  [CrCtl_st] -> Relational Operator22/1
  Constant29/1 -> Relational Operator22/2
  [CrCtl_stOpFunc] -> Relational Operator24/1
  Constant30/1 -> Relational Operator24/2
  Relational Operator22/1 -> Logical Operator23/1
  Relational Operator24/1 -> Logical Operator23/2
  Logical Operator23/1 -> Logical Operator24/1, Logical Operator28/1, Logical Operator27/1, Logical Operator26/1
  Constant31/1 -> TurnOnDelay3/2
  Constant32/1 -> TurnOnDelay3/3
  [GlbDa_vXFlt] -> Relational Operator27/2, Relational Operator26/2, Relational Operator25/2, Relational Operator23/1
  CrCtl_vDes/1 -> Add1/1, Add3/1, Product/1, Add2/1
  Constant33/1 -> Add1/2
  Add1/1 -> Relational Operator23/2
  Relational Operator23/1 -> Logical Operator25/1, TurnOnDelay3/1
  Logical Operator25/1 -> Logical Operator24/2
  Constant34/1 -> Add2/2
  Add2/1 -> Relational Operator25/1
  Bit Clear21/1 -> Switch22/3
  Bit Set21/1 -> Switch22/1
  Switch23/1 -> Bit Clear21/1, Bit Set21/1
  Relational Operator25/1 -> Logical Operator26/2
  Constant35/1 -> Add3/2
  Add3/1 -> Relational Operator26/1
  Relational Operator26/1 -> Logical Operator27/2
  Bit Clear22/1 -> Switch23/3
  Bit Set22/1 -> Switch23/1
  Switch24/1 -> Bit Set22/1, Bit Clear22/1
  Bit Clear23/1 -> Switch24/3
  Bit Set23/1 -> Switch24/1
  Switch25/1 -> Bit Clear23/1, Bit Set23/1
  Constant36/1 -> Product/2
  Relational Operator27/1 -> Logical Operator28/2
  Product/1 -> Relational Operator27/1
  Bit Clear24/1 -> Switch25/3
  Bit Set24/1 -> Switch25/1
  Switch26/1 -> Bit Clear24/1, Bit Set24/1
  Bit Clear25/1 -> Switch26/3
  Bit Set25/1 -> Switch26/1
  Switch27/1 -> Bit Clear25/1, Bit Set25/1
  Bit Clear26/1 -> Switch27/3
  Switch28/1 -> Bit Clear26/1, Bit Set26/1
  Bit Set26/1 -> Switch27/1
  Bit Clear27/1 -> Switch28/3
  Switch29/1 -> Bit Clear27/1, Bit Set27/1
  Bit Set27/1 -> Switch28/1
  Bit Clear28/1 -> Switch29/3
  Switch32/1 -> Bit Clear28/1, Bit Set28/1
  Bit Set28/1 -> Switch29/1
  Gbx_bGearShftActv/1 -> Relational Operator28/1
  Constant37/1 -> Relational Operator28/2
  WESDem_stCrCtlShutOff/1 -> Relational Operator29/1
  Constant38/1 -> Relational Operator29/2
  HndBrk_stDebVal/1 -> Relational Operator30/1
  Constant39/1 -> Relational Operator30/2
  EBrk_stPreSelMode/1 -> Data Type Conversion2/1
  Constant40/1 -> Relational Operator31/2
  Constant41/1 -> Relational Operator32/2
  Relational Operator31/1 -> Logical Operator29/1
  Relational Operator32/1 -> Logical Operator29/2
  APP_r/1 -> Chk_DrvDemActv_Hi/4(APP_r), Chk_DrvDemActv/4(APP_r)
  CoETS_stInrDesBrk/1 -> Terminator1/1
  VehMot_rTrqDfftl/1 -> Chk_DrvDemActv/5(VehMot_rTrqDfftl)
  PT_rTrq/1 -> Chk_DrvDemActv/6(PT_rTrq)
  PT_trqLos/1 -> Chk_DrvDemActv/7(PT_trqLos)
  RngMod_trqCrSMin/1 -> Chk_DrvDemActv/8(RngMod_trqCrSMin)
  CoVeh_trqAcs/1 -> Chk_DrvDemActv/9(CoVeh_trqAcs)
  Constant42/1 -> GetBit/2
  Constant43/1 -> GetBit1/2
  Constant44/1 -> GetBit2/2
  Constant45/1 -> GetBit3/2
  Constant46/1 -> GetBit4/2
  Constant47/1 -> GetBit5/2
  GlbDa_stTrqDem/1 -> GetBit/1, GetBit5/1, GetBit4/1, GetBit3/1, GetBit2/1, GetBit1/1
  Constant48/1 -> Relational Operator33/1
  Constant49/1 -> Relational Operator33/2
  Relational Operator33/1 -> Switch31/2
  GetBit/1 -> Logical Operator30/1
  GetBit1/1 -> Logical Operator30/2
  GetBit2/1 -> Switch31/1
  Logical Operator30/1 -> Switch31/3
  Switch31/1 -> Logical Operator31/1
  Constant50/1 -> GetBit6/2
  GetBit6/1 -> Logical Operator32/1
  [SpdGov_trqSet] -> Logical Operator37/2, Relational Operator34/1
  Constant51/1 -> Relational Operator34/2
  Relational Operator34/1 -> Logical Operator32/2
  Logical Operator32/1 -> Logical Operator31/2
  Constant52/1 -> Relational Operator35/2
  [CrCtl_st] -> Relational Operator35/1, Relational Operator36/1
  Relational Operator35/1 -> Logical Operator33/1
  Relational Operator36/1 -> Logical Operator33/2
  Constant53/1 -> Relational Operator36/2
  Logical Operator31/1 -> Logical Operator34/1
  Logical Operator33/1 -> Logical Operator39/1, Logical Operator34/2
  Constant54/1 -> Relational Operator37/1
  Constant55/1 -> Relational Operator37/2
  Relational Operator37/1 -> Switch30/2
  GetBit3/1 -> Logical Operator35/1
  GetBit4/1 -> Logical Operator35/2
  Logical Operator35/1 -> Switch30/3
  GetBit5/1 -> Switch30/1
  Constant56/1 -> GetBit7/2
  Constant57/1 -> GetBit8/2
  CoETS_stTSEATrqSpdReq/1 -> GetBit8/1, GetBit7/1, GetBit6/1
  GetBit7/1 -> Logical Operator36/1
  GetBit8/1 -> Logical Operator36/2
  Logical Operator36/1 -> Logical Operator37/1
  Switch30/1 -> Logical Operator38/1
  Logical Operator37/1 -> Logical Operator38/2
  Logical Operator38/1 -> Logical Operator39/2
  Bit Clear29/1 -> Switch32/3
  Switch33/1 -> Bit Clear29/1, Bit Set29/1
  Bit Set29/1 -> Switch32/1
  Bit Clear30/1 -> Switch33/3
  Switch/1 -> Unit Delay/1, CrCtl_stShOffCon_mp/1
  Bit Set30/1 -> Switch33/1
  Unit Delay/1 -> Bit Clear30/1, Bit Set30/1
  Data Type Conversion2/1 -> Relational Operator32/1, Relational Operator31/1
  Unit Delay1/1 -> Switch9/1
  Relational Operator6/1 -> Logical Operator15/2
  Constant58/1 -> Relational Operator6/2
  Constant59/1 -> Relational Operator38/2
  Logical Operator18/1 -> Switch17/2
  Logical Operator19/1 -> Switch18/2
  Logical Operator20/1 -> Switch19/2
  Logical Operator22/1 -> Switch20/2
  Logical Operator24/1 -> Switch21/2
  Logical Operator26/1 -> Switch22/2
  Logical Operator27/1 -> Switch23/2
  Logical Operator28/1 -> Switch24/2
  Relational Operator28/1 -> Switch25/2
  LLim_stCrCtlShOff/1 -> Switch26/2
  Relational Operator29/1 -> Switch27/2
  Relational Operator30/1 -> Switch28/2
  Logical Operator29/1 -> Switch29/2
  Logical Operator34/1 -> Switch32/2
  Logical Operator39/1 -> Switch33/2
  Logical Operator13/1 -> Switch15/2
  Logical Operator11/1 -> Switch14/2
  Logical Operator10/1 -> Switch13/2
  Logical Operator9/1 -> Switch12/2
  Logical Operator7/1 -> Switch11/2
  Logical Operator5/1 -> Switch10/2
  Constant4/1 -> Switch8/2
  EBC1/VDC1 Shut off conditons/1(Out1) -> Switch7/2
  Constant3/1 -> Switch6/2
  Logical Operator2/1 -> Switch5/2
  Logical Operator1/1 -> Switch4/2
  Logical Operator/1 -> Switch3/2
  Relational Operator2/1 -> Switch2/2
  Relational Operator1/1 -> Switch1/2
  Relational Operator/1 -> Switch/2
  TurnOnDelay3/1 -> Logical Operator25/2

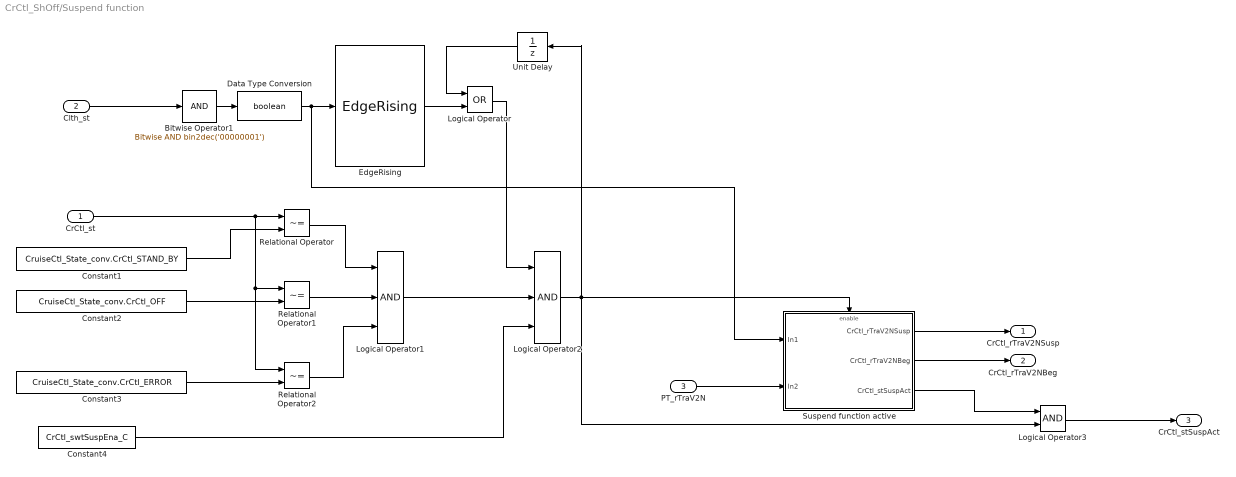
== system CrCtl_ShOff/Suspend function ==
  CrCtl_st : Inport
  Clth_st : Inport  Port=2
  PT_rTraV2N : Inport  Port=3
  Bitwise Operator1 : simulink/Logic and Bit Operations/Bitwise Operator  logicop=AND  UseBitMask=on  BitMask=bin2dec('00000001')  BitMaskRealWorld=Stored Integer
  Constant1 : Constant  Value=CruiseCtl_State_conv.CrCtl_STAND_BY
  Constant2 : Constant  Value=CruiseCtl_State_conv.CrCtl_OFF
  Constant3 : Constant  Value=CruiseCtl_State_conv.CrCtl_ERROR
  Constant4 : Constant  Value=CrCtl_swtSuspEna_C
  Data Type Conversion : DataTypeConversion  OutDataTypeStr=boolean
  EdgeRising : CXLib/EdgeRising
  Logical Operator : Logic  Operator=OR  AllPortsSameDT=off  OutDataTypeStr=boolean
  Logical Operator1 : Logic  Inputs=3  AllPortsSameDT=off  OutDataTypeStr=boolean
  Logical Operator2 : Logic  Inputs=3  AllPortsSameDT=off  OutDataTypeStr=boolean
  Logical Operator3 : Logic  AllPortsSameDT=off  OutDataTypeStr=boolean
  Relational Operator : RelationalOperator  Operator=~=  OutDataTypeStr=boolean  RndMeth=Simplest
  Relational Operator1 : RelationalOperator  Operator=~=  OutDataTypeStr=boolean  RndMeth=Simplest
  Relational Operator2 : RelationalOperator  Operator=~=  OutDataTypeStr=boolean  RndMeth=Simplest
  Suspend function active : Subsystem  TreatAsAtomicUnit=on
  Unit Delay : UnitDelay  SampleTime=-1
  CrCtl_rTraV2NSusp : Outport
  CrCtl_rTraV2NBeg : Outport  Port=2
  CrCtl_stSuspAct : Outport  Port=3
  wires:
  Clth_st/1 -> Bitwise Operator1/1
  Bitwise Operator1/1 -> Data Type Conversion/1
  EdgeRising/1 -> Logical Operator/2
  CrCtl_st/1 -> Relational Operator2/1, Relational Operator1/1, Relational Operator/1
  Constant1/1 -> Relational Operator/2
  Constant2/1 -> Relational Operator1/2
  Constant3/1 -> Relational Operator2/2
  Relational Operator1/1 -> Logical Operator1/2
  Relational Operator/1 -> Logical Operator1/1
  Relational Operator2/1 -> Logical Operator1/3
  Logical Operator1/1 -> Logical Operator2/2
  Constant4/1 -> Logical Operator2/3
  Logical Operator/1 -> Logical Operator2/1
  Logical Operator2/1 -> Logical Operator3/2, Suspend function active/Enable, Unit Delay/1
  PT_rTraV2N/1 -> Suspend function active/2(In2)
  Data Type Conversion/1 -> Suspend function active/1(In1), EdgeRising/1
  Suspend function active/1(CrCtl_rTraV2NSusp) -> CrCtl_rTraV2NSusp/1
  Suspend function active/2(CrCtl_rTraV2NBeg) -> CrCtl_rTraV2NBeg/1
  Logical Operator3/1 -> CrCtl_stSuspAct/1
  Suspend function active/3(CrCtl_stSuspAct) -> Logical Operator3/1
  Unit Delay/1 -> Logical Operator/1

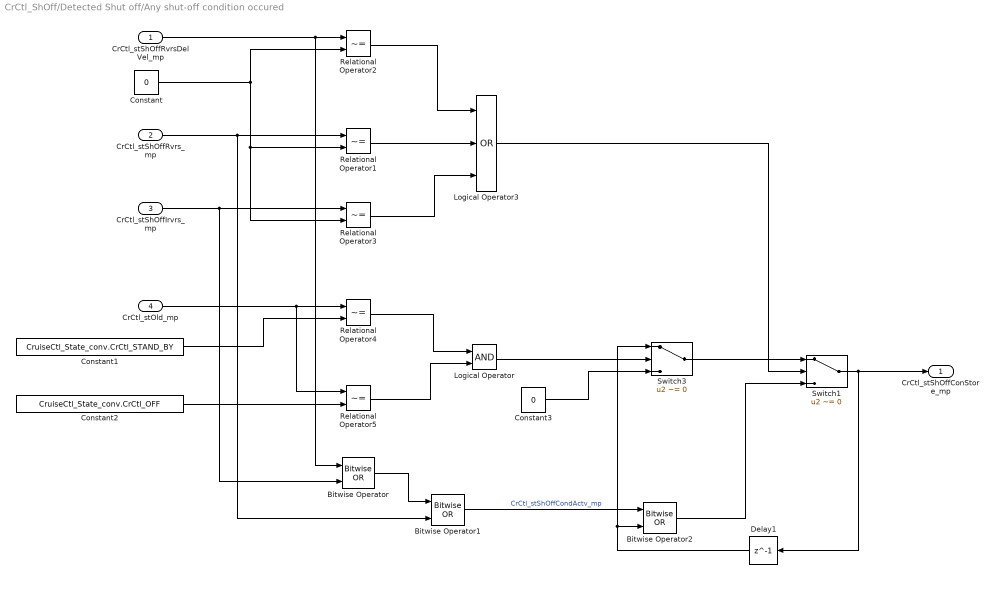
== system CrCtl_ShOff/Detected Shut off/Any shut-off condition occured ==
  CrCtl_stShOffRvrsDelVel_mp : Inport
  CrCtl_stShOffRvrs_mp : Inport  Port=2
  CrCtl_stShOffIrvrs_mp : Inport  Port=3
  CrCtl_stOld_mp : Inport  Port=4
  Bitwise Operator : simulink/Logic and Bit Operations/Bitwise Operator  logicop=OR  UseBitMask=off  NumInputPorts=2  BitMask=bin2dec('11011001')  BitMaskRealWorld=Stored Integer
  Bitwise Operator1 : simulink/Logic and Bit Operations/Bitwise Operator  logicop=OR  UseBitMask=off  NumInputPorts=2  BitMask=bin2dec('11011001')  BitMaskRealWorld=Stored Integer
  Bitwise Operator2 : simulink/Logic and Bit Operations/Bitwise Operator  logicop=OR  UseBitMask=off  NumInputPorts=2  BitMask=bin2dec('11011001')  BitMaskRealWorld=Stored Integer
  Constant : Constant  Value=0  OutDataTypeStr=uint16
  Constant1 : Constant  Value=CruiseCtl_State_conv.CrCtl_STAND_BY
  Constant2 : Constant  Value=CruiseCtl_State_conv.CrCtl_OFF
  Constant3 : Constant  Value=0  OutDataTypeStr=int16
  Delay1 : Delay  DelayLength=1  InitialCondition=0
  Logical Operator : Logic  AllPortsSameDT=off  OutDataTypeStr=boolean
  Logical Operator3 : Logic  Operator=OR  Inputs=3  AllPortsSameDT=off  OutDataTypeStr=boolean
  Relational Operator{1..5} (5 alike) : RelationalOperator  Operator=~=  OutDataTypeStr=boolean  RndMeth=Simplest
  Switch1 : Switch  Criteria=u2 ~= 0
  Switch3 : Switch  Criteria=u2 ~= 0
  CrCtl_stShOffConStore_mp : Outport
  wires:
  CrCtl_stShOffRvrsDelVel_mp/1 -> Bitwise Operator/1, Relational Operator2/1
  Constant/1 -> Relational Operator2/2, Relational Operator3/2, Relational Operator1/2
  CrCtl_stShOffRvrs_mp/1 -> Bitwise Operator1/2, Relational Operator1/1
  CrCtl_stShOffIrvrs_mp/1 -> Bitwise Operator/2, Relational Operator3/1
  Constant1/1 -> Relational Operator4/2
  CrCtl_stOld_mp/1 -> Relational Operator5/1, Relational Operator4/1
  Constant2/1 -> Relational Operator5/2
  Bitwise Operator/1 -> Bitwise Operator1/1
  Relational Operator4/1 -> Logical Operator/1
  Relational Operator5/1 -> Logical Operator/2
  Relational Operator1/1 -> Logical Operator3/2
  Relational Operator2/1 -> Logical Operator3/1
  Relational Operator3/1 -> Logical Operator3/3
  Logical Operator/1 -> Switch3/2
  Constant3/1 -> Switch3/3
  Bitwise Operator1/1 -> Bitwise Operator2/1  "CrCtl_stShOffCondActv_mp"
  Switch3/1 -> Switch1/1
  Logical Operator3/1 -> Switch1/2
  Bitwise Operator2/1 -> Switch1/3
  Delay1/1 -> Switch3/1, Bitwise Operator2/2
  Switch1/1 -> CrCtl_stShOffConStore_mp/1, Delay1/1
